simulink model "Main_Simulink"  (R2013b)
settings: Solver=ode4  StartTime=0.0  StopTime=3.5  FixedStep=0.01  RelTol=1e-3
values from neighbouring files (symbols this model uses):
  An = [-1.02   0.905 ... (first row only)    [Incertezas.m]    (also in Main.m; Teste_paper_Robusto_ITA_My_Analisis.m)
  Bn = [ -0.0215 ... (first row only)    [Incertezas.m]    (also in Main.m; Teste_paper_Robusto_ITA_My_Analisis.m)
  Cn = [    0  57.295 ... (first row only)    [Incertezas.m]    (also in Main.m; Teste_paper_Robusto_ITA_My_Analisis.m)
  Dn = [     0 ... (first row only)    [Incertezas.m]    (also in Main.m; Teste_paper_Robusto_ITA_My_Analisis.m)
  Ki = T.Blocks.ki.Value    [Main.m]
  Kp = T.Blocks.kp.Value    [Main.m]
  Kq = tf(kq,1)    [Custo.m]    (also in Incertezas.m; Main.m = T.Blocks.kq.Value; RestricoesNaoLineares.m; Teste_paper_Robusto_ITA_My_Analisis.m)
settings Model: Creator=Eduardo  LastModifiedBy=Eduardo

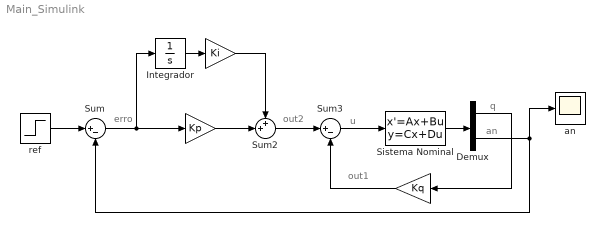
== system Main_Simulink ==
  note: u
  note: out2
  note: out1
  note: erro
  note: an
  note: q
  " " : Gain  Gain=Kq
  "  " : Gain  Gain=Kp
  "   " : Gain  Gain=Ki
  Demux : Demux  Outputs=2
  Integrador : Integrator
  Sistema Nominal : StateSpace  A=An  B=Bn  C=Cn  D=Dn  X0=0
  Sum : Sum  Inputs=|+-
  Sum2 : Sum  Inputs=++|
  Sum3 : Sum  Inputs=|+-
  "an " : Scope
  ref : Step  Time=0  SampleTime=0
  wires:
  Sistema Nominal/1 -> Demux/1
  ref/1 -> Sum/1
  Demux/2 -> Sum/2, "an "/1
  Demux/1 -> " "/1
  Sum/1 -> "  "/1, Integrador/1
  Integrador/1 -> "   "/1
  "   "/1 -> Sum2/1
  "  "/1 -> Sum2/2
  " "/1 -> Sum3/2
  Sum2/1 -> Sum3/1
  Sum3/1 -> Sistema Nominal/1
